simulink model "ASM_Traffic_V2X_Complete_Model_2"  (R2019a)
settings: Solver=ode1  StartTime=SIM.tstart.v  StopTime=Inf  FixedStep=SIM.StepSize.v  RelTol=1e-3
PostLoadFcn:
  | if any(exist('dsrtsu_mdlpostloadfcn', 'file') ~= 0), dsrtsu_mdlpostloadfcn('Execute', bdroot); end
  | try, asm_mdl_postloadfcn(bdroot, 'UpdateModel', 2200); catch, disp(lasterr); end,
undefined symbols (not defined in the file): _SensorPnts_1, _SensorPnts_13, _SensorPnts_17, _SensorPnts_21, _SensorPnts_25, _SensorPnts_29, _SensorPnts_33, _SensorPnts_37, _SensorPnts_41, _SensorPnts_45, _SensorPnts_49, _SensorPnts_5, _SensorPnts_53, _SensorPnts_57, _SensorPnts_9, _to_, CPT, G5A, ITS, MDL, rad, s_to_rpm, SIM
libraries: simulink x169, ASM_VehicleDynamics_lib x126, ASM_Traffic_lib x83, ASM_Utils_lib x49, mdbs x45, ASM_Environment_lib x17, dspindex x12, dsaV2xLibraryAux x10, dsmpblib x6, dsaV2xAsn1Library x4, dsaV2xLibrary x4, ASM_BrakeHydraulics_lib x4
(part 36 of 36)

== system ASM_Traffic_V2X_Complete_Model_2/IO/I//O_Subsystem/Bus Configuration (1) - Out/Simulated ECUs/DrivekitCAN/Drivekit/RX/PDUs/CHASSIS_CONTROL_COMMAND/left_signal/ISignal Value ==
  ISignal Value : Inport
  Term_left_signal Value : Terminator
  _ISignal Value_ : BusSelector  OutputSignals=left_signal Value
  wires:
  ISignal Value/1 -> _ISignal Value_/1  "ISignal Value"
  _ISignal Value_/1 -> Term_left_signal Value/1  "<left_signal Value>"

== system ASM_Traffic_V2X_Complete_Model_2/IO/I//O_Subsystem/Bus Configuration (1) - Out/Simulated ECUs/DrivekitCAN/Drivekit/RX/PDUs/CHASSIS_CONTROL_COMMAND/rear_wiper/ISignal Value ==
  ISignal Value : Inport
  Term_rear_wiper Value : Terminator
  _ISignal Value_ : BusSelector  OutputSignals=rear_wiper Value
  wires:
  ISignal Value/1 -> _ISignal Value_/1  "ISignal Value"
  _ISignal Value_/1 -> Term_rear_wiper Value/1  "<rear_wiper Value>"

== system ASM_Traffic_V2X_Complete_Model_2/IO/I//O_Subsystem/Bus Configuration (1) - Out/Simulated ECUs/DrivekitCAN/Drivekit/RX/PDUs/CHASSIS_CONTROL_COMMAND/right_signal/ISignal Value ==
  ISignal Value : Inport
  Term_right_signal Value : Terminator
  _ISignal Value_ : BusSelector  OutputSignals=right_signal Value
  wires:
  ISignal Value/1 -> _ISignal Value_/1  "ISignal Value"
  _ISignal Value_/1 -> Term_right_signal Value/1  "<right_signal Value>"

== system ASM_Traffic_V2X_Complete_Model_2/IO/I//O_Subsystem/Bus Configuration (1) - Out/Simulated ECUs/DrivekitCAN/Drivekit/RX/PDUs/CHASSIS_CONTROL_COMMAND/vin/ISignal Value ==
  ISignal Value : Inport
  Term_vin Value : Terminator
  _ISignal Value_ : BusSelector  OutputSignals=vin Value
  wires:
  ISignal Value/1 -> _ISignal Value_/1  "ISignal Value"
  _ISignal Value_/1 -> Term_vin Value/1  "<vin Value>"

== system ASM_Traffic_V2X_Complete_Model_2/IO/I//O_Subsystem/Bus Configuration (1) - Out/Simulated ECUs/DrivekitCAN/Drivekit/RX/PDUs/STEERING_ANGLE_COMMAND/steering_angle_cmd_angle/ISignal Value ==
  ISignal Value : Inport
  Term_steering_angle_cmd_angle Value : Terminator
  _ISignal Value_ : BusSelector  OutputSignals=steering_angle_cmd_angle Value
  wires:
  ISignal Value/1 -> _ISignal Value_/1  "ISignal Value"
  _ISignal Value_/1 -> Term_steering_angle_cmd_angle Value/1  "<steering_angle_cmd_angle Value>"

== system ASM_Traffic_V2X_Complete_Model_2/IO/I//O_Subsystem/Bus Configuration (1) - Out/Simulated ECUs/DrivekitCAN/Drivekit/RX/PDUs/STEERING_ANGLE_COMMAND/steering_angle_cmd_flags/ISignal Value ==
  ISignal Value : Inport
  Term_steering_angle_cmd_flags Value : Terminator
  _ISignal Value_ : BusSelector  OutputSignals=steering_angle_cmd_flags Value
  wires:
  ISignal Value/1 -> _ISignal Value_/1  "ISignal Value"
  _ISignal Value_/1 -> Term_steering_angle_cmd_flags Value/1  "<steering_angle_cmd_flags Value>"

== system ASM_Traffic_V2X_Complete_Model_2/IO/I//O_Subsystem/Bus Configuration (1) - Out/Simulated ECUs/DrivekitCAN/Drivekit/RX/PDUs/STEERING_ANGLE_COMMAND/steering_angle_cmd_max_velocity/ISignal Value ==
  ISignal Value : Inport
  Term_steering_angle_cmd_max_velocity Value : Terminator
  _ISignal Value_ : BusSelector  OutputSignals=steering_angle_cmd_max_velocity Value
  wires:
  ISignal Value/1 -> _ISignal Value_/1  "ISignal Value"
  _ISignal Value_/1 -> Term_steering_angle_cmd_max_velocity Value/1  "<steering_angle_cmd_max_velocity Value>"

== system ASM_Traffic_V2X_Complete_Model_2/IO/I//O_Subsystem/Bus Configuration (1) - Out/Simulated ECUs/DrivekitCAN/Drivekit/RX/PDUs/STEERING_DISABLE/steering_disable_magic/ISignal Value ==
  ISignal Value : Inport
  Term_steering_disable_magic Value : Terminator
  _ISignal Value_ : BusSelector  OutputSignals=steering_disable_magic Value
  wires:
  ISignal Value/1 -> _ISignal Value_/1  "ISignal Value"
  _ISignal Value_/1 -> Term_steering_disable_magic Value/1  "<steering_disable_magic Value>"

== system ASM_Traffic_V2X_Complete_Model_2/IO/I//O_Subsystem/Bus Configuration (1) - Out/Simulated ECUs/DrivekitCAN/Drivekit/RX/PDUs/STEERING_ENABLE/steering_enable_magic/ISignal Value ==
  ISignal Value : Inport
  Term_steering_enable_magic Value : Terminator
  _ISignal Value_ : BusSelector  OutputSignals=steering_enable_magic Value
  wires:
  ISignal Value/1 -> _ISignal Value_/1  "ISignal Value"
  _ISignal Value_/1 -> Term_steering_enable_magic Value/1  "<steering_enable_magic Value>"

== system ASM_Traffic_V2X_Complete_Model_2/IO/I//O_Subsystem/Bus Configuration (1) - Out/Simulated ECUs/DrivekitCAN/Drivekit/RX/PDUs/STEERING_TORQUE_COMMAND/steering_command_magic/ISignal Value ==
  ISignal Value : Inport
  Term_steering_command_magic Value : Terminator
  _ISignal Value_ : BusSelector  OutputSignals=steering_command_magic Value
  wires:
  ISignal Value/1 -> _ISignal Value_/1  "ISignal Value"
  _ISignal Value_/1 -> Term_steering_command_magic Value/1  "<steering_command_magic Value>"

== system ASM_Traffic_V2X_Complete_Model_2/IO/I//O_Subsystem/Bus Configuration (1) - Out/Simulated ECUs/DrivekitCAN/Drivekit/RX/PDUs/STEERING_TORQUE_COMMAND/steering_torque_command/ISignal Value ==
  ISignal Value : Inport
  Term_steering_torque_command Value : Terminator
  _ISignal Value_ : BusSelector  OutputSignals=steering_torque_command Value
  wires:
  ISignal Value/1 -> _ISignal Value_/1  "ISignal Value"
  _ISignal Value_/1 -> Term_steering_torque_command Value/1  "<steering_torque_command Value>"

== system ASM_Traffic_V2X_Complete_Model_2/IO/I//O_Subsystem/Bus Configuration (1) - Out/Simulated ECUs/DrivekitCAN/Drivekit/RX/PDUs/THROTTLE_COMMAND/throttle_command_magic/ISignal Value ==
  ISignal Value : Inport
  Term_throttle_command_magic Value : Terminator
  _ISignal Value_ : BusSelector  OutputSignals=throttle_command_magic Value
  wires:
  ISignal Value/1 -> _ISignal Value_/1  "ISignal Value"
  _ISignal Value_/1 -> Term_throttle_command_magic Value/1  "<throttle_command_magic Value>"

== system ASM_Traffic_V2X_Complete_Model_2/IO/I//O_Subsystem/Bus Configuration (1) - Out/Simulated ECUs/DrivekitCAN/Drivekit/RX/PDUs/THROTTLE_COMMAND/throttle_pedal_command/ISignal Value ==
  ISignal Value : Inport
  Term_throttle_pedal_command Value : Terminator
  _ISignal Value_ : BusSelector  OutputSignals=throttle_pedal_command Value
  wires:
  ISignal Value/1 -> _ISignal Value_/1  "ISignal Value"
  _ISignal Value_/1 -> Term_throttle_pedal_command Value/1  "<throttle_pedal_command Value>"

== system ASM_Traffic_V2X_Complete_Model_2/IO/I//O_Subsystem/Bus Configuration (1) - Out/Simulated ECUs/DrivekitCAN/Drivekit/RX/PDUs/THROTTLE_DISABLE/throttle_disable_magic/ISignal Value ==
  ISignal Value : Inport
  Term_throttle_disable_magic Value : Terminator
  _ISignal Value_ : BusSelector  OutputSignals=throttle_disable_magic Value
  wires:
  ISignal Value/1 -> _ISignal Value_/1  "ISignal Value"
  _ISignal Value_/1 -> Term_throttle_disable_magic Value/1  "<throttle_disable_magic Value>"

== system ASM_Traffic_V2X_Complete_Model_2/IO/I//O_Subsystem/Bus Configuration (1) - Out/Simulated ECUs/DrivekitCAN/Drivekit/RX/PDUs/THROTTLE_ENABLE/throttle_enable_magic/ISignal Value ==
  ISignal Value : Inport
  Term_throttle_enable_magic Value : Terminator
  _ISignal Value_ : BusSelector  OutputSignals=throttle_enable_magic Value
  wires:
  ISignal Value/1 -> _ISignal Value_/1  "ISignal Value"
  _ISignal Value_/1 -> Term_throttle_enable_magic Value/1  "<throttle_enable_magic Value>"

== matlab function ASM_Traffic_V2X_Complete_Model_2/MDL/Environment/Driver/SteeringWheelAngle_Control/steeringWheeelSelectionFunction ==
  data: clock input; speed input; strAngle output; swaSim input; swaFile input
function strAngle = fcn(clock,speed,swaSim,swaFile)

if (clock>=8 && clock<=15)
    strAngle = swaSim;
    
else if (clock>=25 && clock<=29)
    strAngle = swaSim;
else
    strAngle = 0;
end
end

== matlab function ASM_Traffic_V2X_Complete_Model_2/IO/V2X_Subsystem/CAM-DENM_Message_Generation/Queue_CAM_DENM/MATLAB Function2 ==
  data: cam input; outvector_v2x output; denm input; camEnable input; denmEnable input; z input
function outvector_v2x = fcn(cam,denm,camEnable,denmEnable,z)

if z ==1 && camEnable ==1
    outvector_v2x = cam;

elseif z ==2 && denmEnable == 1
    outvector_v2x = denm;
    
elseif z ==2 && denmEnable == 0
    outvector_v2x = cam;
    
else
    outvector_v2x=denm;
end
end

== matlab function ASM_Traffic_V2X_Complete_Model_2/IO/V2X_Subsystem/Car_Data/Fellow_ID_1/Heading Function ==
  data: u input; y output
function y = fcn(u)
    while (u>360)
        u=u-360;
    end
    
    while (u<-360)
        u=u+360;
    end
y = u;

== matlab function ASM_Traffic_V2X_Complete_Model_2/IO/V2X_Subsystem/CAM-DENM_Message_Generation/Queue_CAM_DENM/MATLAB Function ==
  data: p input; z output
function z = msg_counter(p)

x = rem(p,2);

if x == 1
    
    z = 1;

elseif x == 0
    
    z = 2;

else
   z = 1;
end
    
end

== matlab function ASM_Traffic_V2X_Complete_Model_2/IO/V2X_Subsystem/Car_Data/Fellow_ID_2/Heading Function ==
  data: u input; y output
function y = fcn(u)
    while (u>360)
        u=u-360;
    end
    
    while (u<-360)
        u=u+360;
    end
y = u;

== matlab function ASM_Traffic_V2X_Complete_Model_2/IO/I//O_Subsystem/EgoCar_Data/GPS/MATLAB Function ==
  data: u input; y output
function y = fcn(u)
    while (u>360)
        u=u-360;
    end
    
    while (u<-360)
        u=u+360;
    end
y=u;

end

== matlab function ASM_Traffic_V2X_Complete_Model_2/MDL/Environment/Driver/LateralController/laneNumber ==
  data: u input; laneNumber output
function laneNumber = fcn(u)
%u : Position of the Ego Vehicle on y axis as meters

if (u<=-1.76) && (u >=-6)
    laneNumber = 1;
elseif (u>=-8.7) && (u <=-6)
    laneNumber = 2;
elseif (u<=1.75) && (u >=-1.75)
    laneNumber = 0 ;
else
    laneNumber = 9 ;
end
end

== matlab function ASM_Traffic_V2X_Complete_Model_2/IO/V2X_Subsystem/Car_Data/Fellow_ID_3/Heading Function ==
  data: u input; y output
function y = fcn(u)
    while (u>360)
        u=u-360;
    end
    
    while (u<-360)
        u=u+360;
    end
y = u;

== matlab function ASM_Traffic_V2X_Complete_Model_2/IO/V2X_Subsystem/CAM-DENM_Message_Generation/Queue_CAM/MATLAB Function ==
  data: cam1 input; e1 input; cam2 input; e2 input; cam3 input; e3 input; z input; outvectorcam output
function outvectorcam = fcn(cam1,e1,cam2,e2,cam3,e3,z)


if z ==1 && e1==1
    outvectorcam = cam1;
elseif z ==2 && e2==1
     outvectorcam = cam2;
elseif z==3 && e3==1
    outvectorcam  = cam3;
elseif e1==0 && e2==0 && e3==0
    outvectorcam = cam1 ;
else
    outvectorcam = cam1 ;
end

== matlab function ASM_Traffic_V2X_Complete_Model_2/IO/V2X_Subsystem/CAM-DENM_Message_Generation/Queue_CAM/MATLAB Function1 ==
  data: p input; z output
function z = ornek(p)

x = rem(p,3);

if x == 1
    
    z = 1;

elseif x == 2
    
    z = 2;

else
   z = 3;
end
    
end
